simulink model "Motor_ctrl"  (R2025b)
settings: Solver=ode15s  StopTime=Tend_sim  FixedStep=Ts/10  MaxStep=Tstep  AbsTol=1e-3  EnableMultiTasking=on
InitFcn:
  | if ~exist('flagwp')
  |     tic
  |     init_sim
  | end
  | mex Motor_ctrl.c User_functions/Src/*.c
StopFcn:
  | % if ~exist('flagwp')
  |   elapsed_time=toc
  | % end
  | %plot_out_sim
values from neighbouring files (symbols this model uses):
  accel = 30000    [init_sim.m]
  Bm = 0.02    [init_sim.m]
  Clarke_inv = [1 0;-0.5 sqrt(3)/2;-0.5 -sqrt(3)/2]    [init_sim.m]
  Ctrl_strategy = 1    [init_sim.m]
  Ctrl_type = 3    [init_sim.m]
  dem = 1    [init_sim.m]
  dT = motorModel.SyreDrive.Converter.dT * 1e-6    [init_sim.m]
  EV_mode = 0    [init_sim.m]
  expC = motorModel.IronPMLossMap_dq.expC    [init_sim.m]
  expH = motorModel.IronPMLossMap_dq.expH    [init_sim.m]
  expPM = motorModel.IronPMLossMap_dq.expPM    [init_sim.m]
  Fd0 = interp2(motorModel.FluxMap_dq.Id,motorModel.FluxMap_dq.Iq,motorModel.FluxMap_dq.Fd,0,0)    [init_sim.m]
  fD_pu_norm = motorModel.FluxMapInv_dq.fD_pu_norm    [init_sim.m]
  fD_vct_max = motorModel.FluxMapInv_dq.fD_vct_max    [init_sim.m]
  fD_vct_ref = motorModel.FluxMapInv_dq.fD_vct_ref    [init_sim.m]
  Fm = interp2(Idd,Iqq,Fdd,0,0)    [init_sim.m]
  fQ_pu_norm = motorModel.FluxMapInv_dq.fQ_pu_norm    [init_sim.m]
  fQ_vct_max = motorModel.FluxMapInv_dq.fQ_vct_max    [init_sim.m]
  fQ_vct_ref = motorModel.FluxMapInv_dq.fQ_vct_ref    [init_sim.m]
  HS_ctrl = 1    [init_sim.m]
  Id_dqt = interpn(motorModel.FluxMapInv_dqt.dataF.Fd,motorModel.FluxMapInv_dqt.dataF.Fq,motorModel.FluxMapInv_dqt.dataF.th,motorModel.FluxMapInv_dqt.dataF.Id,Fd_dqt,Fq_dqt,th_dqt,'cubic')    [init_sim.m]
  Id_fe = motorModel.IronPMLossMap_dq.Id    [init_sim.m]
  iD_pu_norm = motorModel.FluxMapInv_dq.iD_pu_norm    [init_sim.m]
  idRef = interp1(abs(MTPA.id+1i*MTPA.iq),MTPA.id,i0)    [init_sim.m]
  InitIntg_d = Fm*cos(th0)    [init_sim.m]
  InitIntg_q = Fm*sin(th0)    [init_sim.m]
  inj_waveform = 1    [init_sim.m]
  Iq_dqt = interpn(motorModel.FluxMapInv_dqt.dataF.Fd,motorModel.FluxMapInv_dqt.dataF.Fq,motorModel.FluxMapInv_dqt.dataF.th,motorModel.FluxMapInv_dqt.dataF.Iq,Fd_dqt,Fq_dqt,th_dqt,'cubic')    [init_sim.m]
  Iq_fe = motorModel.IronPMLossMap_dq.Iq    [init_sim.m]
  iQ_pu_norm = motorModel.FluxMapInv_dq.iQ_pu_norm    [init_sim.m]
  iqRef = interp1(abs(MTPA.id+1i*MTPA.iq),MTPA.iq,i0)    [init_sim.m]
  IronLoss = 1    [init_sim.m]
  J = 2.7    [init_sim.m]
  motorModelType = motorModel.SyreDrive.modelSetup.motorModelType    [init_sim.m]
  n0 = motorModel.IronPMLossMap_dq.n0    [init_sim.m]
  nRef = 1000    [init_sim.m]
  p = motorModel.data.p    [init_sim.m]
  Pfe_c = motorModel.IronPMLossMap_dq.Pfes_c + motorModel.IronPMLossMap_dq.Pfer_c    [init_sim.m]
  Pfe_h = motorModel.IronPMLossMap_dq.Pfes_h + motorModel.IronPMLossMap_dq.Pfer_h    [init_sim.m]
  Ppm = motorModel.IronPMLossMap_dq.Ppm    [init_sim.m]
  Quad_Maps = 2    [init_sim.m]
  Rs = motorModel.data.Rs    [init_sim.m]
  SS_on = 1    [init_sim.m]
  T0 = interp2(motorModel.FluxMap_dq.Id,motorModel.FluxMap_dq.Iq,motorModel.FluxMap_dq.T,idRef,iqRef)    [init_sim.m]
  T_dqt = interpn(motorModel.FluxMapInv_dqt.dataF.Fd,motorModel.FluxMapInv_dqt.dataF.Fq,motorModel.FluxMapInv_dqt.dataF.th,motorModel.FluxMapInv_dqt.dataF.T,Fd_dqt,Fq_dqt,th_dqt,'cubic')    [init_sim.m]
  Tf = 6    [init_sim.m]
  th0 = 0    [init_sim.m]
  th_max = max(motorModel.FluxMapInv_dqt.dataF.th,[],'all')    [init_sim.m]
  th_min = min(motorModel.FluxMapInv_dqt.dataF.th,[],'all')    [init_sim.m]
  Ts = 1/motorModel.SyreDrive.Converter.fPWM    [init_sim.m]
  Tv = 7.1e-6    (= 7.1e-06)    [init_sim.m]
  VDC = motorModel.data.Vdc    [init_sim.m]
undefined symbols (not defined in the file or in its folder): ACloss, eMotor, interpn, J_rot, magnitude, n0_inv
libraries: nesl_utility x31, fl_lib x26, simulink x10, ee_lib x8, eeTransforms x1
(part 1 of 4)
settings Model: SimulationMode=accelerator  Creator=work  LastModifiedBy=Simone Ferrari
settings SolverCC: ZeroCrossAlgorithm=Adaptive  AlgebraicLoopSolver=TrustRegion
settings DataIOCC: FinalStateName=xFinalSim  InitialState=xFinalSim  SaveFormat=Array  SignalLoggingSaveFormat=ModelDataLogs  SaveOutput=off  SignalLogging=off  DSMLogging=off  TimeSaveName=time  SignalLoggingName=sigsOut
settings OptimizationCC: BlockReduction=off  BooleanDataType=off  ExpressionDepthLimit=2147483647.0  InitFltsAndDblsToZero=on  LifeSpan=inf
settings DebuggingCC: SaveWithParameterizedLinksMsg=none  SignalResolutionControl=TryResolveAllWithWarning  IgnoredZcDiagnostic=none  MultiTaskDSMMsg=warning  MultiTaskCondExecSysMsg=none  FcnCallInpInsideContextMsg=warning  UnconnectedInputMsg=warning  UnconnectedOutputMsg=warning  UnconnectedLineMsg=warning  StateNameClashWarn=warning  SFUnexpectedBacktrackingDiag=warning  SFNoUnconditionalDefaultTransitionDiag=warning  SFExecutionAtInitializationDiag=none  ArithmeticOperatorsInVariantConditions=warning
settings HardwareCC: ProdBitPerPointer=32.0  ProdBitPerSizeT=32.0  ProdBitPerPtrDiffT=32.0  ProdLargestAtomicFloat=None  ProdIntDivRoundTo=Undefined  ProdEndianess=Unspecified  ProdWordSize=32.0  ProdHWDeviceType=32-bit Generic  TargetBitPerPointer=64.0  TargetBitPerSizeT=64.0  TargetBitPerPtrDiffT=64.0  TargetLongLongMode=on  TargetIntDivRoundTo=Zero  TargetEndianess=LittleEndian  TargetWordSize=64.0  TargetHWDeviceType=MATLAB Host  ProdEqTarget=off
settings ModelReferenceCC: EnableRefExpFcnMdlSchedulingChecks=on
settings SFSimCC: SimUseLocalCustomCode=off  CustomCodeUndefinedFunction=UseInterfaceOnly
settings RTWCC: RTWUseLocalCustomCode=off  GPUComputeCapability=3.5  DLArmComputeVersion=19.05
settings CodeAppCC: StateflowObjectComments=on
settings GRTTargetCC: TargetFcnLib=ansi_tfl_tmw.mat  TargetLangStandard=C89/C90 (ANSI)  CombineOutputUpdateFcns=off  GRTInterface=on
settings ConfigComp: CovMetricSettings=dw  CovSaveCumulativeToWorkspaceVar=on  CovSaveSingleToWorkspaceVar=on  CovExternalEMLEnable=off  CovSFcnEnable=off

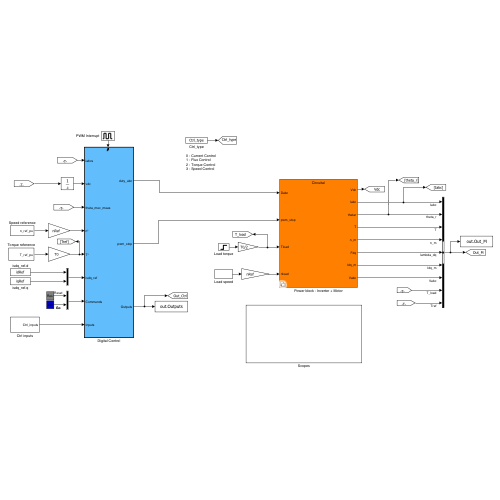
[thumbnail: Simulink's stored preview of the top-level diagram]
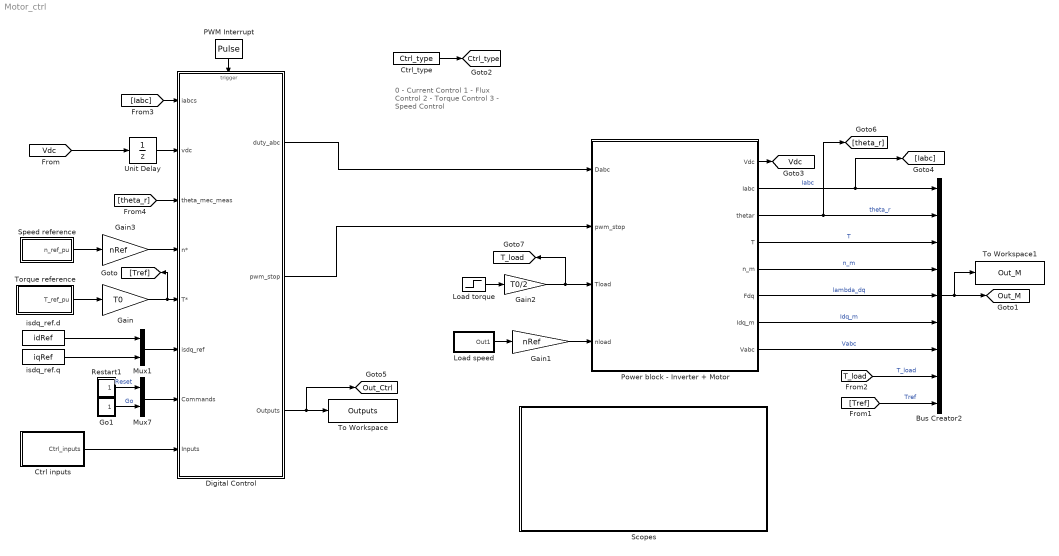
== system Motor_ctrl ==
  note: 0 - Current Control
      | 1 - Flux Control
      | 2 - Torque Control
      | 3 - Speed Control
  Bus Creator2 : BusCreator  Inputs=9
  Ctrl inputs : Subsystem
  Ctrl_type : Constant  Value=Ctrl_type
  Digital Control : Subsystem  TreatAsAtomicUnit=on
  Gain : Gain  Gain=T0
  Gain1 : Gain  Gain=nRef
  Gain2 : Gain  Gain=T0/2
  Gain3 : Gain  Gain=nRef
  Go1 : Subsystem
  Load speed : Subsystem
  Load torque : Step  Time=0.6  SampleTime=0
  Mux1 : Mux  Inputs=2
  Mux7 : Mux  Inputs=2
  PWM Interrupt : DiscretePulseGenerator  PulseType=Time based  Period=Ts  PulseWidth=50
  Power block - Inverter + Motor : Subsystem  Variant=on
  Restart1 : Subsystem
  Scopes : Subsystem
  Speed reference : Subsystem
  To Workspace : ToWorkspace  VariableName=Outputs  SaveFormat=Timeseries  SampleTime=-1
      settings: Decimation=n_dec
  To Workspace1 : ToWorkspace  VariableName=Out_M  SaveFormat=Timeseries  SampleTime=-1
      settings: Decimation=n_dec
  Torque reference : Subsystem
  Unit Delay : UnitDelay  SampleTime=-1
  isdq_ref.d : Constant  Value=idRef
  isdq_ref.q : Constant  Value=iqRef
  tag scope: Ctrl_type=global, Out_Ctrl=global, Out_M=global, T_load=global, Vdc=global
  wires:
  Gain/1 -> [Tref], Digital Control/5(T*)
  Digital Control/2(pwm_stop) -> Power block - Inverter + Motor/2(pwm_stop)
  Unit Delay/1 -> Digital Control/2(vdc)
  isdq_ref.d/1 -> Mux1/1
  Restart1/1(Res) -> Mux7/1  "Reset"
  isdq_ref.q/1 -> Mux1/2
  PWM Interrupt/1 -> Digital Control/Trigger
  Gain3/1 -> Digital Control/4(n*)
  Digital Control/3(Outputs) -> [Out_Ctrl], To Workspace/1
  Digital Control/1(duty_abc) -> Power block - Inverter + Motor/1(Dabc)
  Mux7/1 -> Digital Control/7(Commands)
  Ctrl_type/1 -> [Ctrl_type]
  Gain2/1 -> Power block - Inverter + Motor/3(Tload), [T_load]
  Load torque/1 -> Gain2/1
  Mux1/1 -> Digital Control/6(isdq_ref)
  Go1/1(Go) -> Mux7/2  "Go"
  Speed reference/1(n_ref_pu) -> Gain3/1
  [T_load] -> Bus Creator2/8  "T_load"
  Power block - Inverter + Motor/2(Iabc) -> Bus Creator2/1, [Iabc]  "Iabc"
  Power block - Inverter + Motor/7(Idq_m) -> Bus Creator2/6  "Idq_m"
  Power block - Inverter + Motor/5(n_m) -> Bus Creator2/4  "n_m"
  Power block - Inverter + Motor/3(thetar) -> Bus Creator2/2, [theta_r]  "theta_r"
  Power block - Inverter + Motor/4(T) -> Bus Creator2/3  "T"
  [Tref] -> Bus Creator2/9  "Tref"
  Bus Creator2/1 -> To Workspace1/1, [Out_M]
  Power block - Inverter + Motor/6(Fdq) -> Bus Creator2/5  "lambda_dq"
  Power block - Inverter + Motor/8(Vabc) -> Bus Creator2/7  "Vabc"
  Gain1/1 -> Power block - Inverter + Motor/4(nload)
  Torque reference/1(T_ref_pu) -> Gain/1
  Ctrl inputs/1(Ctrl_inputs) -> Digital Control/8(Inputs)
  Power block - Inverter + Motor/1(Vdc) -> [Vdc]
  [Vdc] -> Unit Delay/1
  [Iabc] -> Digital Control/1(iabcs)
  [theta_r] -> Digital Control/3(theta_mec_meas)
  Load speed/1(Out1) -> Gain1/1

== system Motor_ctrl/Ctrl inputs ==
  Constant1 : Constant  Value=Fm
  Constant10 : Constant  Value=Quad_Maps
  Constant2 : Constant  Value=th0
  Constant3 : Constant  Value=Ctrl_strategy
  Constant5 : Constant  Value=SS_on
  Constant6 : Constant  Value=inj_waveform
  Constant7 : Constant  Value=HS_ctrl
  Constant8 : Constant  Value=dem
  Constant9 : Constant  Value=accel
  Mux9 : Mux  Inputs=10
  Ctrl_inputs : Outport
  wires:
  Constant7/1 -> Mux9/5
  Constant10/1 -> Mux9/8
  Constant3/1 -> Mux9/2
  Constant6/1 -> Mux9/3
  Constant1/1 -> Mux9/9
  Constant8/1 -> Mux9/4
  Constant9/1 -> Mux9/7
  Constant2/1 -> Mux9/10
  Constant5/1 -> Mux9/6
  [Ctrl_type] -> Mux9/1
  Mux9/1 -> Ctrl_inputs/1

== system Motor_ctrl/Digital Control ==
  iabcs : Inport
  vdc : Inport  Port=2
  theta_mec_meas : Inport  Port=3
  n* : Inport  Port=4
  T* : Inport  Port=5
  isdq_ref : Inport  Port=6
  Commands : Inport  Port=7
  Inputs : Inport  Port=8
  Trigger : TriggerPort  VariantControl=(inherit)
  Bus Creator : BusCreator  Inputs=42
  Control S-Function : S-Function  FunctionName=Motor_ctrl  SFunctionDeploymentMode=off  EnableBusSupport=off
  Demux1 : Demux  Outputs=2
  Demux2 : Demux  Outputs=45
  Mux : Mux  Inputs=9
  Mux1 : Mux  Inputs=3
  Unit Delay : UnitDelay  SampleTime=-1
  duty_abc : Outport
  pwm_stop : Outport  Port=2
  Outputs : Outport  Port=3
  wires:
  Mux/1 -> Control S-Function/1
  vdc/1 -> Mux/2
  theta_mec_meas/1 -> Mux/3
  Control S-Function/1 -> Unit Delay/1
  n*/1 -> Mux/4
  Mux1/1 -> Bus Creator/1, duty_abc/1  "duty_abc"
  Demux1/1 -> Mux/7  "Reset"
  Demux1/2 -> Mux/8  "Go"
  Commands/1 -> Demux1/1
  isdq_ref/1 -> Mux/6
  Unit Delay/1 -> Demux2/1
  Demux2/1 -> Mux1/1  "duty_a"
  Demux2/2 -> Mux1/2  "duty_b"
  Demux2/3 -> Mux1/3  "duty_c"
  Demux2/4 -> pwm_stop/1
  T*/1 -> Mux/5
  Inputs/1 -> Mux/9
  Bus Creator/1 -> Outputs/1
  Demux2/34 -> Bus Creator/31  "pos_err_HS"
  Demux2/33 -> Bus Creator/30  "pos_err_LS"
  Demux2/32 -> Bus Creator/29  "pos_err_real"
  Demux2/31 -> Bus Creator/28  "pos_err"
  Demux2/30 -> Bus Creator/27  "theta_elt_meas"
  Demux2/29 -> Bus Creator/26  "iC"
  Demux2/28 -> Bus Creator/25  "iB"
  Demux2/27 -> Bus Creator/24  "iA"
  Demux2/26 -> Bus Creator/23  "ldq"
  Demux2/25 -> Bus Creator/22  "lq"
  Demux2/24 -> Bus Creator/21  "ld"
  Demux2/23 -> Bus Creator/20  "n_ctrl"
  Demux2/22 -> Bus Creator/19  "theta_elt"
  Demux2/21 -> Bus Creator/18  "T_ext"
  Demux2/20 -> Bus Creator/17  "lambdaQ_CM"
  Demux2/18 -> Bus Creator/15  "lambdaQ"
  Demux2/19 -> Bus Creator/16  "lambdaD_CM"
  Demux2/17 -> Bus Creator/14  "lambdaD"
  Demux2/16 -> Bus Creator/13  "T_elt"
  Demux2/15 -> Bus Creator/12  "f_w"
  Demux2/14 -> Bus Creator/11  "iq"
  Demux2/13 -> Bus Creator/10  "iq_ref"
  Demux2/12 -> Bus Creator/9  "id"
  Demux2/11 -> Bus Creator/8  "id_ref"
  Demux2/10 -> Bus Creator/7  "isbeta"
  Demux2/9 -> Bus Creator/6  "isalpha"
  Demux2/8 -> Bus Creator/5  "vq_ref"
  Demux2/7 -> Bus Creator/4  "vd_ref"
  Demux2/6 -> Bus Creator/3  "wr"
  Demux2/5 -> Bus Creator/2  "wr_ref"
  iabcs/1 -> Mux/1
  Demux2/35 -> Bus Creator/32  "lambda_ref"
  Demux2/36 -> Bus Creator/33  "lambda_fbk"
  Demux2/37 -> Bus Creator/34  "iqs_ref"
  Demux2/38 -> Bus Creator/35  "iqs_fbk"
  Demux2/39 -> Bus Creator/36  "delta_max"
  Demux2/40 -> Bus Creator/37  "delta_fbk"
  Demux2/41 -> Bus Creator/38  "i_MTPV"
  Demux2/42 -> Bus Creator/39  "iqs_Lim"
  Demux2/43 -> Bus Creator/40  "vds_ref"
  Demux2/44 -> Bus Creator/41  "vqs_ref"
  Demux2/45 -> Bus Creator/42  "State"

== system Motor_ctrl/Go1 ==
  GO_Down : Step  Time=0.01+4*Ts  SampleTime=0
  GO_Up : Step  Time=0.01  SampleTime=0
  Subtract : Sum  Inputs=+-
  Go : Outport
  wires:
  Subtract/1 -> Go/1
  GO_Up/1 -> Subtract/1
  GO_Down/1 -> Subtract/2

== system Motor_ctrl/Load speed ==
  LoadSpeedRamp : simulink/Sources/Ramp  slope=20  start=0.2  InitialOutput=0
  LoadSpeedSat : Saturate  UpperLimit=1  LowerLimit=-1
  Out1 : Outport
  wires:
  LoadSpeedRamp/1 -> LoadSpeedSat/1
  LoadSpeedSat/1 -> Out1/1

== system Motor_ctrl/Power block - Inverter + Motor ==
  note: 1) Add Subsystem or Model blocks as valid variant choices.
      | 2) You cannot connect blocks at this level. At simulation, connectivity is automatically
      | determined, based on the active variant and port name matching.
  Dabc : Inport
  pwm_stop : Inport  Port=2
  Tload : Inport  Port=3
  nload : Inport  Port=4
  Circuital : Subsystem  VariantControl=strcmp(motorModelType,'Controlled Current Generators (CCG)') || strcmp(motorModelType,'SimScape FEM-based PMSM')
  Noncircuital : Subsystem  VariantControl=strcmp(motorModelType,'Non-Circuital Model (FM)')
  Vdc : Outport
  Iabc : Outport  Port=2
  thetar : Outport  Port=3
  T : Outport  Port=4
  n_m : Outport  Port=5
  Fdq : Outport  Port=6
  Idq_m : Outport  Port=7
  Vabc : Outport  Port=8

== system Motor_ctrl/Restart1 ==
  "DOWN " : Step  Time=10e-3+4*Ts  SampleTime=0
  Subtract : Sum  Inputs=+-
  "UP " : Step  Time=10e-3  SampleTime=0
  Res : Outport
  wires:
  "UP "/1 -> Subtract/1
  "DOWN "/1 -> Subtract/2
  Subtract/1 -> Res/1

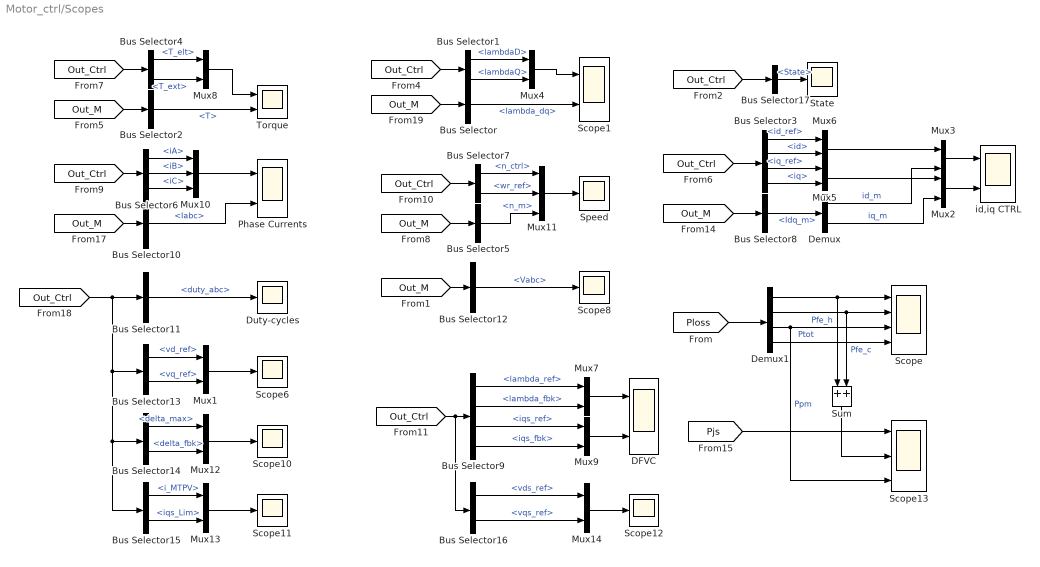
== system Motor_ctrl/Scopes ==
  Bus Selector : BusSelector  OutputSignals=lambda_dq
  Bus Selector1 : BusSelector  OutputSignals=lambdaD,lambdaQ
  Bus Selector10 : BusSelector  OutputSignals=Iabc
  Bus Selector11 : BusSelector  OutputSignals=duty_abc
  Bus Selector12 : BusSelector  OutputSignals=Vabc
  Bus Selector13 : BusSelector  OutputSignals=vd_ref,vq_ref
  Bus Selector14 : BusSelector  OutputSignals=delta_max,delta_fbk
  Bus Selector15 : BusSelector  OutputSignals=i_MTPV,iqs_Lim
  Bus Selector16 : BusSelector  OutputSignals=vds_ref,vqs_ref
  Bus Selector17 : BusSelector  OutputSignals=State
  Bus Selector2 : BusSelector  OutputSignals=T
  Bus Selector3 : BusSelector  OutputSignals=id_ref,id,iq_ref,iq
  Bus Selector4 : BusSelector  OutputSignals=T_elt,T_ext
  Bus Selector5 : BusSelector  OutputSignals=n_m
  Bus Selector6 : BusSelector  OutputSignals=iA,iB,iC
  Bus Selector7 : BusSelector  OutputSignals=n_ctrl,wr_ref
  Bus Selector8 : BusSelector  OutputSignals=Idq_m
  Bus Selector9 : BusSelector  OutputSignals=lambda_ref,lambda_fbk,iqs_ref,iqs_fbk
  DFVC : Scope  NumInputPorts=2
      settings: ActiveDisplayYMinimum=-0.016936566680669781  ActiveDisplayYMaximum=0.15242910012602806
  Demux : Demux  Outputs=2
  Demux1 : Demux
  Duty-cycles : Scope
      settings: ActiveDisplayYMinimum=-0.14215802685897236  ActiveDisplayYMaximum=1.1077597187312376
  Mux{1..9,12..14} (12 alike) : Mux  Inputs=2
  Mux10 : Mux  Inputs=3
  Mux11 : Mux  Inputs=3
  Phase Currents : Scope  NumInputPorts=2
      settings: ActiveDisplayYMinimum=-1311.5522096192847  ActiveDisplayYMaximum=1325.5199197219822
  Scope : Scope  NumInputPorts=4
      settings: ActiveDisplayYMinimum=-1  ActiveDisplayYMaximum=1
  Scope1 : Scope  NumInputPorts=2
      settings: ActiveDisplayYMinimum=-1  ActiveDisplayYMaximum=1
  Scope{6,8,10..12} (5 alike) : Scope
      Scope10 settings: ActiveDisplayYMinimum=-1  ActiveDisplayYMaximum=1
      Scope11 settings: ActiveDisplayYMinimum=-125.78182983398435  ActiveDisplayYMaximum=1132.0364685058594
      Scope12 settings: ActiveDisplayYMinimum=-230.93904685974121  ActiveDisplayYMaximum=230.93997764587402
      Scope6 settings: ActiveDisplayYMinimum=-287.14855575561523  ActiveDisplayYMaximum=243.69842147827148
  Scope13 : Scope  NumInputPorts=3
      settings: ActiveDisplayYMinimum=-1  ActiveDisplayYMaximum=1
  Speed : Scope
      settings: ActiveDisplayYMinimum=-450.47500610351551  ActiveDisplayYMaximum=4054.2750549316406  DataLoggingVariableName=ScopeData2
  State : Scope
      settings: ActiveDisplayYMinimum=-0.37499999999999989  ActiveDisplayYMaximum=3.375  DataLoggingVariableName=ScopeData5
  Sum : Sum
  Torque : Scope  NumInputPorts=2
      settings: ActiveDisplayYMinimum=-62.272152420628927  ActiveDisplayYMaximum=554.91717274463247
  id,iq CTRL : Scope  NumInputPorts=2
      settings: ActiveDisplayYMinimum=-1103.0936021552059  ActiveDisplayYMaximum=934.58880271777161
  wires:
  Bus Selector3/2 -> Mux6/2  "<id>"
  [Out_M] -> Bus Selector2/1
  Mux4/1 -> Scope1/1
  [Out_M] -> Bus Selector12/1
  Bus Selector/1 -> Scope1/2  "<lambda_dq>"
  Bus Selector10/1 -> Phase Currents/2  "<Iabc>"
  Bus Selector1/2 -> Mux4/2  "<lambdaQ>"
  Bus Selector3/3 -> Mux5/1  "<iq_ref>"
  Bus Selector3/4 -> Mux5/2  "<iq>"
  Bus Selector4/1 -> Mux8/1  "<T_elt>"
  Mux6/1 -> Mux3/1
  Demux/1 -> Mux3/2  "id_m"
  [Out_M] -> Bus Selector5/1
  Bus Selector1/1 -> Mux4/1  "<lambdaD>"
  Bus Selector6/3 -> Mux10/3  "<iC>"
  Bus Selector6/2 -> Mux10/2  "<iB>"
  [Out_Ctrl] -> Bus Selector6/1
  [Out_Ctrl] -> Bus Selector1/1
  [Out_Ctrl] -> Bus Selector4/1
  Mux5/1 -> Mux2/1
  Bus Selector6/1 -> Mux10/1  "<iA>"
  [Out_Ctrl] -> Bus Selector7/1
  Mux10/1 -> Phase Currents/1
  [Out_M] -> Bus Selector8/1
  Bus Selector3/1 -> Mux6/1  "<id_ref>"
  [Out_Ctrl] -> Bus Selector3/1
  [Out_M] -> Bus Selector10/1
  Bus Selector12/1 -> Scope8/1  "<Vabc>"
  Mux8/1 -> Torque/1
  Bus Selector8/1 -> Demux/1  "<Idq_m>"
  Demux/2 -> Mux2/2  "iq_m"
  Bus Selector11/1 -> Duty-cycles/1  "<duty_abc>"
  Mux3/1 -> id,iq CTRL/1
  Mux2/1 -> id,iq CTRL/2
  [Out_M] -> Bus Selector/1
  Mux11/1 -> Speed/1
  Demux1/1 -> Sum/1, Scope/1  "Pfe_h"
  Demux1/2 -> Sum/2, Scope/2  "Pfe_c"
  Demux1/4 -> Scope/4  "Ptot"
  Demux1/3 -> Scope13/3, Scope/3  "Ppm"
  Bus Selector2/1 -> Torque/2  "<T>"
  Bus Selector4/2 -> Mux8/2  "<T_ext>"
  Mux1/1 -> Scope6/1
  Bus Selector13/1 -> Mux1/1  "<vd_ref>"
  Bus Selector13/2 -> Mux1/2  "<vq_ref>"
  [Ploss] -> Demux1/1
  [Out_Ctrl] -> Bus Selector16/1, Bus Selector9/1
  Mux7/1 -> DFVC/1
  Bus Selector9/1 -> Mux7/1  "<lambda_ref>"
  Bus Selector9/2 -> Mux7/2  "<lambda_fbk>"
  Bus Selector9/3 -> Mux9/1  "<iqs_ref>"
  Bus Selector9/4 -> Mux9/2  "<iqs_fbk>"
  Mux9/1 -> DFVC/2
  Bus Selector14/2 -> Mux12/2  "<delta_fbk>"
  Mux12/1 -> Scope10/1
  Bus Selector14/1 -> Mux12/1  "<delta_max>"
  Mux13/1 -> Scope11/1
  Bus Selector15/2 -> Mux13/2  "<iqs_Lim>"
  Bus Selector15/1 -> Mux13/1  "<i_MTPV>"
  Bus Selector7/1 -> Mux11/1  "<n_ctrl>"
  Bus Selector7/2 -> Mux11/2  "<wr_ref>"
  Bus Selector5/1 -> Mux11/3  "<n_m>"
  Bus Selector16/2 -> Mux14/2  "<vqs_ref>"
  Mux14/1 -> Scope12/1
  Bus Selector16/1 -> Mux14/1  "<vds_ref>"
  [Out_Ctrl] -> Bus Selector15/1, Bus Selector14/1, Bus Selector13/1, Bus Selector11/1
  [Pjs] -> Scope13/1
  Sum/1 -> Scope13/2
  [Out_Ctrl] -> Bus Selector17/1
  Bus Selector17/1 -> State/1  "<State>"

== system Motor_ctrl/Speed reference ==
  RefSpeedRamp : simulink/Sources/Ramp  slope=20  start=0.2  InitialOutput=0
  RefSpeedRampSat : Saturate  UpperLimit=1  LowerLimit=-1
  n_ref_pu : Outport
  wires:
  RefSpeedRampSat/1 -> n_ref_pu/1
  RefSpeedRamp/1 -> RefSpeedRampSat/1

== system Motor_ctrl/Torque reference ==
  Constant4 : Constant  Value=EV_mode
  EV mode Vs test bench : Switch  Criteria=u2 > Threshold  Threshold=0.5  SaturateOnIntegerOverflow=off  InputSameDT=off
  Step : Step  Time=0.05  SampleTime=0
  Step1 : Step  Time=0.15  SampleTime=0
  Step2 : Step  Time=0.8  After=-2  SampleTime=0
  Sum : Sum
  T_ref_pu : Outport
  wires:
  Constant4/1 -> EV mode Vs test bench/2
  Step/1 -> EV mode Vs test bench/1
  EV mode Vs test bench/1 -> T_ref_pu/1
  Sum/1 -> EV mode Vs test bench/3
  Step2/1 -> Sum/2
  Step1/1 -> Sum/1

== system Motor_ctrl/Power block - Inverter + Motor/Circuital ==
  Dabc : Inport
  pwm_stop : Inport  Port=2
  Tload : Inport  Port=3
  nload : Inport  Port=4
  Inverter Model : Subsystem
  Motor model : Subsystem  Variant=on
  Vdc : Outport
  Iabc : Outport  Port=2
  thetar : Outport  Port=3
  T : Outport  Port=4
  n_m : Outport  Port=5
  Fdq : Outport  Port=6
  Idq_m : Outport  Port=7
  Vabc : Outport  Port=8
  wires:
  Inverter Model/1(Vdc) -> Vdc/1
  Tload/1 -> Motor model/1(Tload)
  nload/1 -> Motor model/2(nload)
  Dabc/1 -> Inverter Model/1(Dabc)
  pwm_stop/1 -> Inverter Model/2(pwm_stop)
  Motor model/1(Iabc) -> Inverter Model/3(Iabc), Iabc/1  "Iabc"
  Motor model/2(thetar) -> thetar/1  "theta_r"
  Motor model/3(T) -> T/1  "T"
  Motor model/4(n_m) -> n_m/1  "n_m"
  Motor model/5(Fdq) -> Fdq/1  "lambda_dq"
  Motor model/6(Idq_m) -> Idq_m/1  "Idq_m"
  Motor model/7(Vabc) -> Vabc/1  "Vabc"
  connections:
  Inverter Model/RConn1 -- Motor model/LConn1
  Inverter Model/RConn2 -- Motor model/LConn2
  Inverter Model/RConn3 -- Motor model/LConn3

== system Motor_ctrl/Power block - Inverter + Motor/Noncircuital ==
  Dabc : Inport
  pwm_stop : Inport  Port=2
  Tload : Inport  Port=3
  nload : Inport  Port=4
  FM : Subsystem
  Inverter Model : Subsystem  VariantControl=Choice
  Vdc : Outport
  Iabc : Outport  Port=2
  thetar : Outport  Port=3
  T : Outport  Port=4
  n_m : Outport  Port=5
  Fdq : Outport  Port=6
  Idq_m : Outport  Port=7
  Vabc : Outport  Port=8
  wires:
  FM/4(n_m) -> n_m/1  "n_m"
  FM/1(Iabc) -> Iabc/1, Inverter Model/3(Iabc)  "Iabc"
  FM/3(Tm) -> T/1  "T_m"
  FM/5(Fdq) -> Fdq/1  "lambda_dq"
  FM/2(thetar) -> thetar/1  "theta_r"
  FM/6(Idq_m) -> Idq_m/1  "Idq_m"
  pwm_stop/1 -> Inverter Model/2(pwm_stop)
  Tload/1 -> FM/1(Tload)
  Dabc/1 -> Inverter Model/1(Dabc)
  FM/7(Vabc) -> Vabc/1  "Vabc"
  nload/1 -> FM/2(nload)
  Inverter Model/1(Vdc) -> Vdc/1
  Inverter Model/2(Va) -> FM/3(A)
  Inverter Model/3(Vb) -> FM/4(B)
  Inverter Model/4(Vc) -> FM/5(C)

== system Motor_ctrl/Power block - Inverter + Motor/Circuital/Inverter Model ==
  Dabc : Inport
  pwm_stop : Inport  Port=2
  Iabc : Inport  Port=3
  " " : Fcn  Expr=1-u(1)
  Converter (Three-Phase) : ee_lib/Semiconductors & Converters/Converters/Converter (Three-Phase)  port_option=ee.enum.threePhasePort.expanded  fidelity_option=ee.enum.converters.fidelity.detailed  device_type=ee.enum.converters.switchingdevice.ideal  showThermalPort=false  K=0  Vth=0.001 V  Vgt=1 V  Vgt_off=-1 V  Ih=1 A  Vf=0.001 V  Ron=Rd Ohm  Rds=0.001 Ohm  Goff=1e-4 1/Ohm  Eon_scalar=22.86e-3 J  Eoff_scalar=17.14e-3 J  Eoff_natural_commutation=10e-3 J  Voff=300 V  Iout_scalar=600 A  onCurrentMeasDelay=0 s  useCurrentFromPreviousCycle=false  useVoltageFromPreviousCycle=false  diode_param=ee.enum.converters.protectiondiode.nodynamics  diode_Vf=0.8 V  diode_Ron=1e-4 Ohm  diode_Goff=1e-5 1/Ohm  diode_C=50 nF  diode_iRM=-235 A  diode_iF=300 A  diode_idot=-50 A/us  diode_trr_param=ee.enum.converters.diodetrr.trr_factor  diode_trr_factor=3  diode_trr=15 us  diode_Qrr=1500 s*uA  diode_rec_loss_model=ee.enum.diode.reverseRecoveryModel.fixed  diode_ErecVal=0 J  diode_scaleWithIandV=false  diode_ErecMat=zeros(2, 3) J  diode_TjrecVec=[298.15, 398.15] K  diode_IfrecVec=[.1, 1, 10] A  diode_IrecVal=10 A  diode_VrecVal=10 V  diode_tFilter=1 / 1000 / 100 s  thermal_network_parameterization=ee.enum.thermalNetworkTopology.external  Rth=[.08, .5] K/W  Rth_Cauer=[.08, .1, .5] K/W  Rth_Foster=[.08, .14, .22, .16] K/W  thermal_mass_parameterization=ee.enum.thermalNetwork.timeconstant  thermal_mass=[.01, .5] J/K  thermal_mass_Cauer=[.01, .1, .5] J/K  thermal_mass_Foster=[.001, .005, .05, .5] J/K  thermal_time_constant=[.001, .2] s  thermal_time_constant_Cauer=[.001, .1, .2] s  thermal_time_constant_Foster=[7e-05, .0007, .01, .08] s  thermal_mass_initial_temperatures=[25, 25] degC  thermal_mass_initial_temperatures_Cauer=[25, 25, 25] degC  junction_thermal_mass=0.01 J/K  Tvec_initial_Foster=[25, 25, 25, 25] degC  snubber_type=ee.enum.converters.snubber.exclude  Cs=1e-7 F  Rs=0.1 Ohm  Vce_loss=[0, 150, 300] V
  Demux : Demux  Outputs=6
  Electrical Reference : fl_lib/Electrical/Electrical Elements/Electrical Reference
  Inverter Commands : Subsystem  Variant=on
  PS-Simulink Converter : nesl_utility/PS-Simulink Converter  PhysicalDomain=network_engine_domain  SubClassName=ps_output  LeftPortType=input  RightPortType=output  PseudoPeriodic=off  Frequencies=[]  VectorFormat=1-D array  Unit=inherit  AffineConversion=off
  Simulink-PS Converter{,1..5} (6 alike) : nesl_utility/Simulink-PS Converter  PhysicalDomain=network_engine_domain  SubClassName=ps_input  LeftPortType=input  RightPortType=output  PseudoPeriodic=off  Frequencies=[]  NoiseDistribution=none  NoiseParameters=[]  Unit=1  AffineConversion=off  FilteringAndDerivatives=provide  SimscapeFilterOrder=1  InputFilterTimeConstant=0.001  UdotUserProvided=0
  Six-Pulse Gate Multiplexer : ee_lib/Semiconductors & Converters/Converters/Six-Pulse Gate Multiplexer  port_option=ee.enum.controlport.ps
  Solver Configuration : nesl_utility/Solver Configuration  PhysicalDomain=network_engine_domain  SubClassName=solver  LeftPortType=input  RightPortType=generic  Tones=[]  Harmonics=[]  SimulateNoise=off  Profile=off  UseLocalSampling=off  EnableSwitchedLinearOptims=on  FrequencyDomain=off  UseCCode=off  RelTol=0.001  AbsTol=1e-06  MinStep=1e-09  ToWorkspace=off  RevertToSquareIcSolve=off  NumHomotopyIterations=100  PhasorMode=off  PhasorModeNumHarmonics=1  ConsistencySolver=NEWTON_FTOL  CanonicalOrdering=UNORDERED  OptimizeIntermediates=UNOPTIMIZED  IndexReductionMethod=DerivativeReplacement  DoDC=off  ResidualTolerance=1e-09  ConsistencyTolSource=GLOBAL  ConsistencyAbsTol=0.001  ConsistencyRelTol=0.001  ConsistencyTolFactor=0.001  UseLocalSolver=off  LocalSolverChoice=NE_BACKWARD_EULER_ADVANCER  ResolveIndetEquations=on  FunctionEvalNumThread=1  LocalSolverSampleTime=Ts/10  DoFixedCost=off  MaxNonlinIter=3  MaxModeIter=2  ComputeImpulses=off  ImpulseIterations=2  LinearAlgebra=auto  LinearAlgebraNumThread=0  EquationFormulation=NE_TIME_EF  DelaysMemoryBudget=1024  AutomaticFiltering=on  FilteringTimeConstant=0.001  PartitionStorageMethod=AS_NEEDED  PartitionMemoryBudget=1024  PartitionMethod=ROBUST  MultibodyUseLocalSolver=off  MultibodyLocalSolverChoice=ODE1  MultibodyLocalSolverSampleTime=0.001
  Voltage Sensor : fl_lib/Electrical/Electrical Sensors/Voltage Sensor
  Voltage Source : ee_lib/Sources/Voltage Source  dc_voltage=0.5*VDC V  ac_voltage=0 V  ac_shift=0 rad  ac_frequency=60 Hz  noise_mode=0  PSD=0 V^2/Hz  sample_time=1e-3 s  repeatability=1  user_seed=0  auto_seed=676943032  i_specify=off  i_priority=None  i=0 A  i_nominal_specify=off  i_nominal_value=1  i_nominal_unit=A  v_specify=off  v_priority=None  v=0 V  v_nominal_specify=off  v_nominal_value=1  v_nominal_unit=V
  Voltage Source1 : ee_lib/Sources/Voltage Source  dc_voltage=0.5*VDC V  ac_voltage=0 V  ac_shift=0 rad  ac_frequency=60 Hz  noise_mode=0  PSD=0 V^2/Hz  sample_time=1e-3 s  repeatability=1  user_seed=0  auto_seed=4168664255  i_specify=off  i_priority=None  i=0 A  i_nominal_specify=off  i_nominal_value=1  i_nominal_unit=A  v_specify=off  v_priority=None  v=0 V  v_nominal_specify=off  v_nominal_value=1  v_nominal_unit=V
  A : PMIOPort  Side=Right
  B : PMIOPort  Port=2  Side=Right
  C : PMIOPort  Port=3  Side=Right
  Vdc : Outport
  wires:
  Iabc/1 -> Inverter Commands/3(iABC)
  Demux/3 -> Simulink-PS Converter2/1
  Demux/4 -> Simulink-PS Converter3/1
  Demux/5 -> Simulink-PS Converter4/1
  Demux/6 -> Simulink-PS Converter5/1
  Demux/1 -> Simulink-PS Converter/1
  Demux/2 -> Simulink-PS Converter1/1
  " "/1 -> Inverter Commands/2(Enable)
  PS-Simulink Converter/1 -> Vdc/1
  Dabc/1 -> Inverter Commands/1(Dabc)
  Inverter Commands/1(G) -> Demux/1
  pwm_stop/1 -> " "/1
  connections:
  Simulink-PS Converter/RConn1 -- Six-Pulse Gate Multiplexer/LConn1
  Simulink-PS Converter3/RConn1 -- Six-Pulse Gate Multiplexer/LConn4
  Solver Configuration/RConn1 -- Converter (Three-Phase)/RConn1 -- Voltage Sensor/LConn1 -- Voltage Source/LConn1
  Simulink-PS Converter4/RConn1 -- Six-Pulse Gate Multiplexer/LConn5
  Simulink-PS Converter2/RConn1 -- Six-Pulse Gate Multiplexer/LConn3
  Simulink-PS Converter1/RConn1 -- Six-Pulse Gate Multiplexer/LConn2
  Simulink-PS Converter5/RConn1 -- Six-Pulse Gate Multiplexer/LConn6
  Voltage Source1/RConn1 -- Converter (Three-Phase)/RConn2 -- Voltage Sensor/RConn2
  Voltage Source/RConn1 -- Voltage Source1/LConn1 -- Electrical Reference/LConn1
  Six-Pulse Gate Multiplexer/RConn1 -- Converter (Three-Phase)/LConn1
  A/RConn1 -- Converter (Three-Phase)/LConn2
  Converter (Three-Phase)/LConn3 -- B/RConn1
  Converter (Three-Phase)/LConn4 -- C/RConn1
  PS-Simulink Converter/LConn1 -- Voltage Sensor/RConn1

== system Motor_ctrl/Power block - Inverter + Motor/Circuital/Motor model ==
  note: 1) Add Subsystem or Model blocks as valid variant choices.
      | 2) You cannot connect blocks at this level. At simulation, connectivity is automatically
      | determined, based on the active variant and port name matching.
  Tload : Inport
  nload : Inport  Port=2
  CCG model : Subsystem  VariantControl=strcmp(motorModelType,'Controlled Current Generators (CCG)')
  SimScape FEM-based PMSM : Subsystem  VariantControl=strcmp(motorModelType,'SimScape FEM-based PMSM')
  A : PMIOPort  Side=Left
  B : PMIOPort  Port=2  Side=Left
  C : PMIOPort  Port=3  Side=Left
  Iabc : Outport
  thetar : Outport  Port=2
  T : Outport  Port=3
  n_m : Outport  Port=4
  Fdq : Outport  Port=5
  Idq_m : Outport  Port=6
  Vabc : Outport  Port=7

== system Motor_ctrl/Power block - Inverter + Motor/Noncircuital/FM ==
  Tload : Inport
  nload : Inport  Port=2
  A : Inport  Port=3
  B : Inport  Port=4
  C : Inport  Port=5
  Mechanical equations : Subsystem
  Motor Model : Subsystem
  Terminator1 : Terminator
  Unit Delay : UnitDelay  SampleTime=-1
  Iabc : Outport
  thetar : Outport  Port=2
  Tm : Outport  Port=3
  n_m : Outport  Port=4
  Fdq : Outport  Port=5
  Idq_m : Outport  Port=6
  Vabc : Outport  Port=7
  wires:
  Mechanical equations/3(thetar) -> Motor Model/2(theta_r), Unit Delay/1
  Motor Model/3(Fdq) -> Fdq/1
  B/1 -> Motor Model/4(B)
  Motor Model/1(Tm) -> Mechanical equations/2(Tm), Tm/1
  Mechanical equations/2(Pmec_out) -> Terminator1/1
  Unit Delay/1 -> thetar/1
  nload/1 -> Mechanical equations/3(RPM)
  Tload/1 -> Mechanical equations/1(Tload)
  Motor Model/5(Vabc) -> Vabc/1
  Mechanical equations/1(n_m) -> Motor Model/1(n_m), n_m/1
  Motor Model/2(Iabc) -> Iabc/1
  Motor Model/4(Idq_m) -> Idq_m/1
  C/1 -> Motor Model/5(C)
  A/1 -> Motor Model/3(A)

== system Motor_ctrl/Power block - Inverter + Motor/Noncircuital/Inverter Model ==
  Dabc : Inport
  pwm_stop : Inport  Port=2
  Iabc : Inport  Port=3
  " " : Fcn  Expr=1-u(1)
  Constant : Constant  Value=VDC
  Demux : Demux  Outputs=3
  Inverter Commands : Subsystem  Variant=on
  Vdc : Outport
  Va : Outport  Port=2
  Vb : Outport  Port=3
  Vc : Outport  Port=4
  wires:
  Iabc/1 -> Inverter Commands/3(iABC)
  pwm_stop/1 -> " "/1
  " "/1 -> Inverter Commands/2(Enable)
  Dabc/1 -> Inverter Commands/1(Dabc)
  Demux/3 -> Vc/1
  Demux/2 -> Vb/1
  Demux/1 -> Va/1
  Inverter Commands/1(Vabc) -> Demux/1
  Constant/1 -> Vdc/1

== system Motor_ctrl/Power block - Inverter + Motor/Circuital/Inverter Model/Inverter Commands ==
  note: 1) Add Subsystem or Model blocks as valid variant choices.
      | 2) You cannot connect blocks at this level. At simulation, connectivity is automatically
      | determined, based on the active variant and port name matching.
  Dabc : Inport
  Enable : Inport  Port=2
  iABC : Inport  Port=3
  Duty : Subsystem  VariantControl=InvModel==0
  PWM : Subsystem  VariantControl=InvModel==1
  G : Outport

== system Motor_ctrl/Power block - Inverter + Motor/Circuital/Motor model/CCG model ==
  Tload : Inport
  nload : Inport  Port=2
  Mechanical equations : Subsystem
  Motor Model : Subsystem
  A : PMIOPort  Side=Left
  B : PMIOPort  Port=2  Side=Left
  C : PMIOPort  Port=3  Side=Left
  Iabc : Outport
  thetar : Outport  Port=2
  T : Outport  Port=3
  n_m : Outport  Port=4
  Fdq : Outport  Port=5
  Idq_m : Outport  Port=6
  Vabc : Outport  Port=7
  wires:
  Mechanical equations/1(n_m) -> Motor Model/1(n_m), n_m/1
  Motor Model/3(Fdq) -> Fdq/1
  Motor Model/5(Vabc) -> Vabc/1
  Motor Model/4(Idq_m) -> Idq_m/1
  Motor Model/1(Te) -> Mechanical equations/2(Te)
  Motor Model/2(Iabc) -> Iabc/1
  Mechanical equations/2(thetar) -> thetar/1, Motor Model/2(theta_r)
  nload/1 -> Mechanical equations/3(RPM)
  Tload/1 -> Mechanical equations/1(Tload)
  Mechanical equations/3(T) -> T/1
  connections:
  B/RConn1 -- Motor Model/LConn2
  C/RConn1 -- Motor Model/LConn3
  A/RConn1 -- Motor Model/LConn1

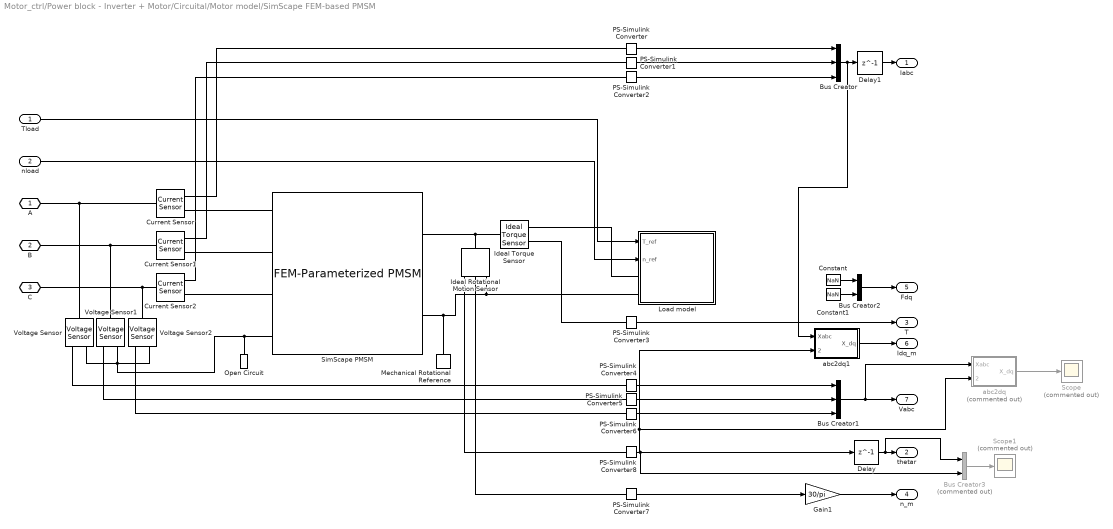
== system Motor_ctrl/Power block - Inverter + Motor/Circuital/Motor model/SimScape FEM-based PMSM ==
  Tload : Inport
  nload : Inport  Port=2
  Bus Creator : BusCreator  Inputs=3
  Bus Creator1 : BusCreator  Inputs=3
  Bus Creator2 : BusCreator  Inputs=2
  Bus Creator3 : BusCreator  Commented=on  Inputs=2
  Constant : Constant  Value=NaN
  Constant1 : Constant  Value=NaN
  Current Sensor : fl_lib/Electrical/Electrical Sensors/Current Sensor
  Current Sensor1 : fl_lib/Electrical/Electrical Sensors/Current Sensor
  Current Sensor2 : fl_lib/Electrical/Electrical Sensors/Current Sensor
  Delay : Delay  DelayLength=1  InitialCondition=0
  Delay1 : Delay  DelayLength=1  InitialCondition=0
  Gain1 : Gain  Gain=30/pi
  Ideal Rotational Motion Sensor : fl_lib/Mechanical/Mechanical Sensors/Ideal Rotational Motion Sensor  reference=foundation.enum.MeasurementReference.difference  acceleration_port=false  velocity_port=true  position_port=true  wrap_angle=true  offset=0 rad
  Ideal Torque Sensor : fl_lib/Mechanical/Mechanical Sensors/Ideal Torque Sensor
  Load model : Subsystem  Variant=on
  Mechanical Rotational Reference : fl_lib/Mechanical/Rotational Elements/Mechanical Rotational Reference
  Open Circuit : fl_lib/Electrical/Electrical Elements/Open Circuit  v_specify=off  v_priority=None  v=0 V  v_nominal_specify=off  v_nominal_value=1  v_nominal_unit=V
  PS-Simulink Converter{,1..8} (9 alike) : nesl_utility/PS-Simulink Converter  PhysicalDomain=network_engine_domain  SubClassName=ps_output  LeftPortType=input  RightPortType=output  PseudoPeriodic=off  Frequencies=[]  VectorFormat=inherit  Unit=inherit  AffineConversion=off
  Scope : Scope  Commented=on
  Scope1 : Scope  Commented=on
  SimScape PMSM : ee_lib/Electromechanical/Permanent Magnet/FEM-Parameterized PMSM  parameterization=1  winding_type=ee.enum.statorconnection.wye  iVec=[-2, 0, 2] A  xVec=[0, 20, 40, 60] deg  dfluxdiMatrix=0.0002 * ones(3, 4) Wb/A  dfluxdxMatrix=[0, -.16, .16, 0; 0, -.16, .16, 0; 0, -.16, .16, 0] Wb/rad  calculate_torque_matrix=1  TorqueMatrix=zeros(3, 3, 3, 4) N*m  idVec1=[-200, 0, 200] A  iqVec1=[-200, 0, 200] A  LdMatrix=0.0002 * ones(3, 3) H  LqMatrix=0.0002 * ones(3, 3) H  PmMatrix=0.1 * ones(3, 3) Wb  interp_method=simscape.enum.interpolation.linear  N=6  Rs=interp1(ACloss.n,ACloss.Rac,0) Ohm  Ms=0.00002 H  L0=eMotor.L0 H  loss_param=ee.enum.fem_motor.ironLossesExtended.tabulated3D  losses_oc=[0, 0, 0] W  losses_sc=[0, 0, 0] W  f_losses=60 Hz  Isc_losses=95 A  Inertia=eMotor.J kg*m^2  lam=0 N*m*s/rad  i_d_specify=on  i_d_priority=None  i_d=0 A  i_d_nominal_specify=off  i_d_nominal_value=1  i_d_nominal_unit=A  i_q_specify=on  i_q_priority=None  i_q=0 A  i_q_nominal_specify=off  i_q_nominal_value=1  i_q_nominal_unit=A  torque_specify=on  torque_priority=None  torque=interpn(eMotor.Id,eMotor.Iq,eMotor.th,eMotor.T,0,0,0) N*m  torque_nominal_specify=off  torque_nominal_value=1  torque_nominal_unit=N*m  angular_velocity_specify=on  angular_velocity_priority=High  angular_velocity=0 rpm  angular_velocity_nominal_specify=off  angular_velocity_nominal_value=1  angular_velocity_nominal_unit=rpm  angular_position_specify=on  angular_position_priority=High  angular_position=0 deg  angular_position_nominal_specify=off  angular_position_nominal_value=1  angular_position_nominal_unit=deg  alpha=3.93e-3 1/K  alpha_flux=-0.001 1/K  Tmeas=298.15 K  stator_thermal_mass=100 J/K  stator_initial_temperatures=[298.15, 298.15, 298.15] K  rotor_thermal_mass=200 J/K  rotor_initial_temperature=298.15 K  Rm_percent_rotor=90  Rd_percent_rotor=30  idVec=[-200, 0, 200] A  iqVec=[-200, 0, 200] A  dfluxAdiaMatrix3D=zeros(3, 3, 4) Wb/A  dfluxAdibMatrix3D=zeros(3, 3, 4) Wb/A  dfluxAdicMatrix3D=zeros(3, 3, 4) Wb/A  dfluxAdxMatrix3D=zeros(3, 3, 4) Wb/rad  TorqueMatrix3D=zeros(3, 3, 4) N*m  iaVec=[-200, 0, 200] A  ibVec=[-200, 0, 200] A  icVec=[-200, 0, 200] A  dfluxAdiaMatrix=zeros(3, 3, 3, 4) Wb/A  dfluxAdibMatrix=zeros(3, 3, 3, 4) Wb/A  dfluxAdicMatrix=zeros(3, 3, 3, 4) Wb/A  dfluxAdxMatrix=zeros(3, 3, 3, 4) Wb/rad  param_dq0=ee.enum.fem_motor.fluxTabulationOption.DQcartesian  winding_type_dq0=ee.enum.statorconnection.wye  expose_neutral_port=ee.enum.fem_motor.exposeNeutralPort.yes  nPolePairs=eMotor.p  parks_type=ee.enum.fem_motor.parksType.QleadsD_AphaseToDaxis  idVec2=eMotor.Id A  iqVec2=eMotor.Iq A  magVec2=[0, 100, 200] A  betaVec2=[-180, -90, 0, 90, 180] deg  xVec2=eMotor.th deg  fluxD_dq0=eMotor.Fd Wb  fluxQ_dq0=eMotor.Fq Wb  fluxA_dq0=zeros(3, 3, 7) Wb  Torque_dq0=eMotor.T N*m  fluxD_IBX=zeros(3, 5, 7) Wb  fluxQ_IBX=zeros(3, 5, 7) Wb  fluxA_IBX=zeros(3, 5, 7) Wb  Torque_IBX=zeros(3, 5, 7) N*m  rotorLossCoeff_k_h_DQ=zeros(3, 3) W/Hz  rotorLossCoeff_k_J_DQ=zeros(3, 3) W/Hz^2  rotorLossCoeff_k_ex_DQ=zeros(3, 3) W/Hz^(3/2)  rotorLossCoeff_k_h_IB=zeros(3, 5) W/Hz  rotorLossCoeff_k_J_IB=zeros(3, 5) W/Hz^2  rotorLossCoeff_k_ex_IB=zeros(3, 5) W/Hz^(3/2)  statorLossCoeff_k_h_DQ=zeros(3, 3) W/Hz  statorLossCoeff_k_J_DQ=zeros(3, 3) W/Hz^2  statorLossCoeff_k_ex_DQ=zeros(3, 3) W/Hz^(3/2)  statorLossCoeff_k_h_IB=zeros(3, 5) W/Hz  statorLossCoeff_k_J_IB=zeros(3, 5) W/Hz^2  statorLossCoeff_k_ex_IB=zeros(3, 5) W/Hz^(3/2)  wVec=eMotor.ironLoss.n rpm  rotorLossTable_DQ=eMotor.ironLoss.Pfer W  statorLossTable_DQ=eMotor.ironLoss.Pfes W  rotorLossTable_IB=zeros(3, 5, 2) W  statorLossTable_IB=zeros(3, 5, 2) W  electrical_torque_before_iron_losses_specify=off  electrical_torque_before_iron_losses_priority=None  electrical_torque_before_iron_losses=0 N*m  electrical_torque_before_iron_losses_nominal_specify=off  electrical_torque_before_iron_losses_nominal_value=1  electrical_torque_before_iron_losses_nominal_unit=N*m  Qrotor_specify=off  Qrotor_priority=None  Qrotor=0 J/s  Qrotor_nominal_specify=off  Qrotor_nominal_value=1  Qrotor_nominal_unit=J/s  Qstator_specify=off  Qstator_priority=None  Qstator=0 J/s  Qstator_nominal_specify=off  Qstator_nominal_value=1  Qstator_nominal_unit=J/s
  Voltage Sensor : fl_lib/Electrical/Electrical Sensors/Voltage Sensor
  Voltage Sensor1 : fl_lib/Electrical/Electrical Sensors/Voltage Sensor
  Voltage Sensor2 : fl_lib/Electrical/Electrical Sensors/Voltage Sensor
  abc2dq : Subsystem  Commented=on
  abc2dq1 : Subsystem
  A : PMIOPort  Side=Left
  B : PMIOPort  Port=2  Side=Left
  C : PMIOPort  Port=3  Side=Left
  Iabc : Outport
  thetar : Outport  Port=2
  T : Outport  Port=3
  n_m : Outport  Port=4
  Fdq : Outport  Port=5
  Idq_m : Outport  Port=6
  Vabc : Outport  Port=7
  wires:
  PS-Simulink Converter1/1 -> Bus Creator/2
  Delay/1 -> Bus Creator3/1, thetar/1
  PS-Simulink Converter3/1 -> T/1
  PS-Simulink Converter7/1 -> Gain1/1
  PS-Simulink Converter4/1 -> Bus Creator1/1
  abc2dq1/1(X_dq) -> Idq_m/1
  Constant1/1 -> Bus Creator2/2
  PS-Simulink Converter/1 -> Bus Creator/1
  Gain1/1 -> n_m/1
  Constant/1 -> Bus Creator2/1
  Bus Creator1/1 -> abc2dq/1(Xabc), Vabc/1
  Delay1/1 -> Iabc/1
  PS-Simulink Converter5/1 -> Bus Creator1/2
  PS-Simulink Converter2/1 -> Bus Creator/3
  abc2dq/1(X_dq) -> Scope/1
  Bus Creator2/1 -> Fdq/1
  Bus Creator3/1 -> Scope1/1
  Bus Creator/1 -> abc2dq1/1(Xabc), Delay1/1
  PS-Simulink Converter6/1 -> Bus Creator1/3
  PS-Simulink Converter8/1 -> Bus Creator3/2, Delay/1, abc2dq1/2(theta_r), abc2dq/2(theta_r)
  Tload/1 -> Load model/1(T_ref)
  nload/1 -> Load model/2(n_ref)
  connections:
  C/RConn1 -- Voltage Sensor2/LConn1 -- Current Sensor2/LConn1
  A/RConn1 -- Voltage Sensor/LConn1 -- Current Sensor/LConn1
  Ideal Rotational Motion Sensor/LConn1 -- SimScape PMSM/RConn1 -- Ideal Torque Sensor/LConn1
  B/RConn1 -- Voltage Sensor1/LConn1 -- Current Sensor1/LConn1
  Voltage Sensor/RConn1 -- PS-Simulink Converter4/LConn1
  Current Sensor1/RConn2 -- SimScape PMSM/LConn2
  PS-Simulink Converter3/LConn1 -- Ideal Torque Sensor/RConn2
  Voltage Sensor1/RConn1 -- PS-Simulink Converter5/LConn1
  PS-Simulink Converter1/LConn1 -- Current Sensor1/RConn1
  PS-Simulink Converter/LConn1 -- Current Sensor/RConn1
  Ideal Rotational Motion Sensor/RConn2 -- PS-Simulink Converter7/LConn1
  Current Sensor2/RConn2 -- SimScape PMSM/LConn3
  PS-Simulink Converter8/LConn1 -- Ideal Rotational Motion Sensor/RConn3
  PS-Simulink Converter6/LConn1 -- Voltage Sensor2/RConn1
  PS-Simulink Converter2/LConn1 -- Current Sensor2/RConn1
  Current Sensor/RConn2 -- SimScape PMSM/LConn1
  Voltage Sensor/RConn2 -- Open Circuit/LConn1 -- SimScape PMSM/LConn4 -- Voltage Sensor1/RConn2 -- Voltage Sensor2/RConn2
  SimScape PMSM/RConn2 -- Mechanical Rotational Reference/LConn1 -- Ideal Rotational Motion Sensor/RConn1 -- Load model/LConn2
  Load model/LConn1 -- Ideal Torque Sensor/RConn1

== system Motor_ctrl/Power block - Inverter + Motor/Noncircuital/FM/Mechanical equations ==
  Tload : Inport
  Tm : Inport  Port=2
  RPM : Inport  Port=3
  Constant : Constant  Value=Tf
  Constant1 : Constant  Value=Tv
  Delay One Step1 : Delay  DelayLength=1
  Delay One Step2 : Delay  DelayLength=1
  Gain1 : Gain  Gain=30/pi
  Gain2 : Gain  Gain=Bm  SaturateOnIntegerOverflow=on  OutDataTypeStr=Inherit: Same as input  ParamDataTypeStr=Inherit: Same as input
  Gain3 : Gain  Gain=1/J  SaturateOnIntegerOverflow=on  OutDataTypeStr=Inherit: Same as input  ParamDataTypeStr=Inherit: Same as input
  Gain4 : Gain  Gain=(2*pi)/60
  Integrator : Integrator  InitialCondition=th0  WrapState=on  WrappedStateUpperValue=2*pi  WrappedStateLowerValue=0
  Integrator1 : Integrator
  Integrator2 : Integrator  InitialCondition=th0  WrapState=on  WrappedStateUpperValue=2*pi  WrappedStateLowerValue=0
  Math Function1 : Math  Operator=magnitude^2  SignedPower=on
  Product : Product  SaturateOnIntegerOverflow=on  OutDataTypeStr=Inherit: Same as first input
  Product3 : Product  SaturateOnIntegerOverflow=on  OutDataTypeStr=Inherit: Same as first input
  Product6 : Product  SaturateOnIntegerOverflow=on  OutDataTypeStr=Inherit: Same as first input
  Sign : Signum  ZeroCross=off
  Sum1 : Sum  SaturateOnIntegerOverflow=on  OutDataTypeStr=Inherit: Same as first input
  Sum4 : Sum  SaturateOnIntegerOverflow=on  OutDataTypeStr=Inherit: Same as first input
  Sum5 : Sum  Inputs=--+  SaturateOnIntegerOverflow=on  OutDataTypeStr=Inherit: Same as first input
  Switch : Switch  Criteria=u2 > Threshold  Threshold=2.5  SaturateOnIntegerOverflow=off  InputSameDT=off
  Switch1 : Switch  Criteria=u2 > Threshold  Threshold=2.5  SaturateOnIntegerOverflow=off  InputSameDT=off
  n_m : Outport
  Pmec_out : Outport  Port=2  VectorParamsAs1DForOutWhenUnconnected=off
  thetar : Outport  Port=3
  wires:
  Gain3/1 -> Integrator1/1
  Gain2/1 -> Sum1/2
  Delay One Step2/1 -> Math Function1/1, Sign/1, Gain2/1
  Product6/1 -> Sum1/1
  Sum1/1 -> Sum5/2  "T mech loss"
  Tm/1 -> Delay One Step1/1
  Product/1 -> Pmec_out/1
  Tload/1 -> Sum5/1
  Math Function1/1 -> Product3/2
  Constant1/1 -> Product3/1
  Product3/1 -> Sum4/2
  Constant/1 -> Sum4/1
  Sum5/1 -> Gain3/1
  Sign/1 -> Product6/2
  Sum4/1 -> Product6/1
  Integrator2/1 -> Switch1/3
  Integrator/1 -> Switch1/1
  Switch1/1 -> thetar/1
  Switch/1 -> Gain1/1
  Integrator1/1 -> Integrator/1, Switch/1, Delay One Step2/1, Product/2
  Gain4/1 -> Switch/3, Integrator2/1
  [Ctrl_type] -> Switch/2, Switch1/2
  RPM/1 -> Gain4/1
  Delay One Step1/1 -> Sum5/3, Product/1
  Gain1/1 -> n_m/1

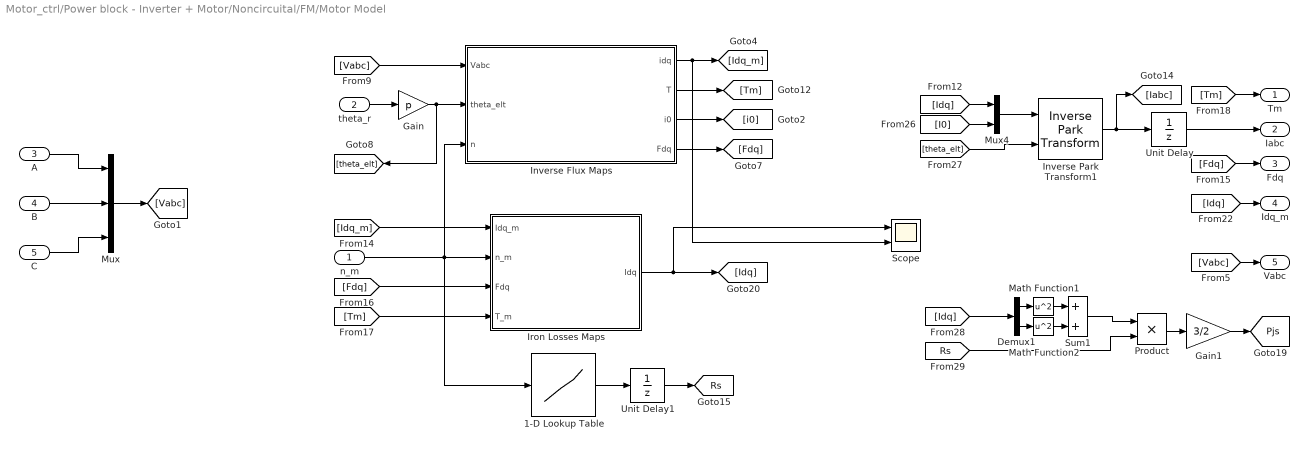
== system Motor_ctrl/Power block - Inverter + Motor/Noncircuital/FM/Motor Model ==
  n_m : Inport
  theta_r : Inport  Port=2
  A : Inport  Port=3
  B : Inport  Port=4
  C : Inport  Port=5
  1-D Lookup Table : Lookup_n-D  NumberOfTableDimensions=1  BreakpointsForDimension1=ACloss.n  Table=ACloss.Rac  InternalRulePriority=Speed  RndMeth=Simplest
  Demux1 : Demux  Outputs=2
  Gain : Gain  Gain=p
  Gain1 : Gain  Gain=3/2
  Inverse Park Transform1 : eeTransforms/Inverse Park Transform  AxisAlignment=D-axis  PowerInvariant=off
  Inverse Flux Maps : Subsystem  Variant=on
  Iron Losses Maps : Subsystem  Variant=on
  Math Function1 : Math  Operator=square
  Math Function2 : Math  Operator=square
  Mux : Mux  Inputs=3
  Mux4 : Mux  Inputs=2
  Product : Product
  Scope : Scope  NumInputPorts=2
  Sum1 : Sum
  Unit Delay : UnitDelay  SampleTime=-1
  Unit Delay1 : UnitDelay  SampleTime=-1
  Tm : Outport
  Iabc : Outport  Port=2
  Fdq : Outport  Port=3
  Idq_m : Outport  Port=4
  Vabc : Outport  Port=5
  tag scope: Pjs=global, Rs=global
  wires:
  Inverse Park Transform1/1 -> [Iabc], Unit Delay/1
  [Idq] -> Idq_m/1
  [Vabc] -> Inverse Flux Maps/1(Vabc)
  [Tm] -> Tm/1
  theta_r/1 -> Gain/1
  [Fdq] -> Fdq/1
  Inverse Flux Maps/2(T) -> [Tm]
  n_m/1 -> Inverse Flux Maps/3(n), 1-D Lookup Table/1, Iron Losses Maps/2(n_m)
  [Fdq] -> Iron Losses Maps/3(Fdq)
  [Tm] -> Iron Losses Maps/4(T_m)
  [Idq_m] -> Iron Losses Maps/1(Idq_m)
  Gain/1 -> [theta_elt], Inverse Flux Maps/2(theta_elt)
  Inverse Flux Maps/3(i0) -> [i0]
  Inverse Flux Maps/4(Fdq) -> [Fdq]
  [Vabc] -> Vabc/1
  [theta_elt] -> Inverse Park Transform1/2
  Mux4/1 -> Inverse Park Transform1/1
  [Idq] -> Mux4/1
  Gain1/1 -> [Pjs]
  Product/1 -> Gain1/1
  [Rs] -> Product/2
  [Idq] -> Demux1/1
  Demux1/1 -> Math Function1/1
  Demux1/2 -> Math Function2/1
  Math Function1/1 -> Sum1/1
  Math Function2/1 -> Sum1/2
  Sum1/1 -> Product/1
  Inverse Flux Maps/1(idq) -> Scope/2, [Idq_m]
  Iron Losses Maps/1(Idq) -> [Idq], Scope/1
  A/1 -> Mux/1
  B/1 -> Mux/2
  C/1 -> Mux/3
  Mux/1 -> [Vabc]
  1-D Lookup Table/1 -> Unit Delay1/1
  Unit Delay/1 -> Iabc/1
  Unit Delay1/1 -> [Rs]
  [I0] -> Mux4/2

== system Motor_ctrl/Power block - Inverter + Motor/Noncircuital/Inverter Model/Inverter Commands ==
  note: 1) Add Subsystem or Model blocks as valid variant choices.
      | 2) You cannot connect blocks at this level. At simulation, connectivity is automatically
      | determined, based on the active variant and port name matching.
  Dabc : Inport
  Enable : Inport  Port=2
  iABC : Inport  Port=3
  Duty : Subsystem  VariantControl=InvModel==0
  PWM : Subsystem  VariantControl=InvModel==1
  Vabc : Outport

== system Motor_ctrl/Power block - Inverter + Motor/Circuital/Inverter Model/Inverter Commands/Duty ==
  Dabc : Inport
  iABC : Inport  Port=2
  Demux : Demux  Outputs=3
  Gain : Gain  Gain=dT/Ts
  Mux14 : Mux  Inputs=6
  Sign : Signum
  Sum : Sum  Inputs=|+-
  X_d1 : Fcn  Expr=1-u(1)
  X_d12 : Fcn  Expr=1-u(1)
  X_d2 : Fcn  Expr=1-u(1)
  G : Outport  VectorParamsAs1DForOutWhenUnconnected=off
  wires:
  iABC/1 -> Sign/1
  Sign/1 -> Gain/1
  Demux/3 -> Mux14/5, X_d2/1
  X_d2/1 -> Mux14/6
  Demux/1 -> X_d12/1, Mux14/1
  Dabc/1 -> Sum/1
  Gain/1 -> Sum/2
  Sum/1 -> Demux/1
  Demux/2 -> Mux14/3, X_d1/1
  X_d1/1 -> Mux14/4
  X_d12/1 -> Mux14/2
  Mux14/1 -> G/1

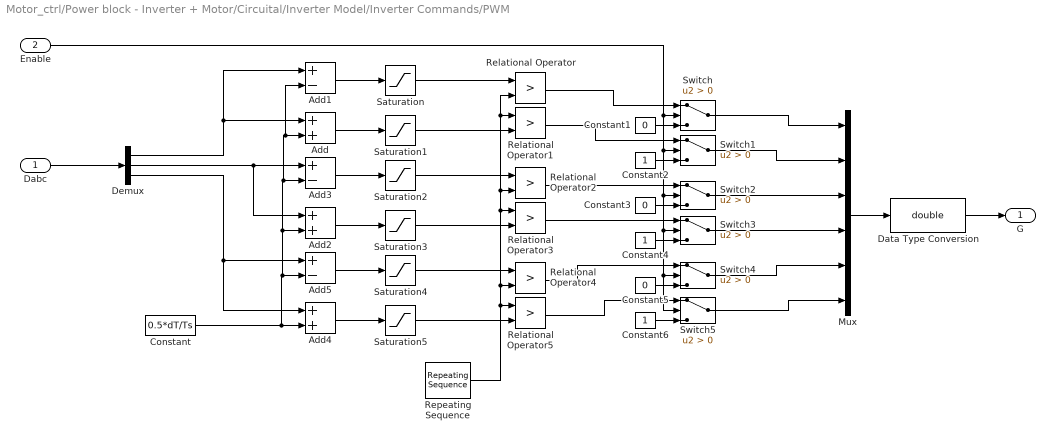
== system Motor_ctrl/Power block - Inverter + Motor/Circuital/Inverter Model/Inverter Commands/PWM ==
  Dabc : Inport
  Enable : Inport  Port=2
  Add : Sum
  Add1 : Sum  Inputs=+-
  Add2 : Sum
  Add3 : Sum  Inputs=+-
  Add4 : Sum
  Add5 : Sum  Inputs=+-
  Constant : Constant  Value=0.5*dT/Ts
  Constant1 : Constant  Value=0
  Constant2 : Constant
  Constant3 : Constant  Value=0
  Constant4 : Constant
  Constant5 : Constant  Value=0
  Constant6 : Constant
  Data Type Conversion : DataTypeConversion  OutDataTypeStr=double  SaturateOnIntegerOverflow=off  RndMeth=Floor
  Demux : Demux  Outputs=3
  Mux : Mux  Inputs=6
  Relational Operator{,1..5} (6 alike) : RelationalOperator  Operator=>  OutDataTypeStr=boolean  RndMeth=Simplest  InputSameDT=off
  Repeating Sequence : simulink/Sources/Repeating Sequence  rep_seq_t=[0 Ts/2 Ts]  rep_seq_y=[1e-6 1-1e-6 1e-6]
  Saturation{,1..5} (6 alike) : Saturate  UpperLimit=1  LowerLimit=0
  Switch{,1..5} (6 alike) : Switch  Criteria=u2 > Threshold  SaturateOnIntegerOverflow=off  InputSameDT=off
  G : Outport
  wires:
  Demux/3 -> Add4/1, Add5/1
  Add4/1 -> Saturation5/1
  Add/1 -> Saturation1/1
  Add5/1 -> Saturation4/1
  Add1/1 -> Saturation/1
  Demux/1 -> Add1/1, Add/1
  Saturation2/1 -> Relational Operator2/1
  Demux/2 -> Add3/1, Add2/1
  Saturation5/1 -> Relational Operator5/2
  Add3/1 -> Saturation2/1
  Add2/1 -> Saturation3/1
  Saturation/1 -> Relational Operator/1
  Saturation4/1 -> Relational Operator4/1
  Saturation1/1 -> Relational Operator1/2
  Saturation3/1 -> Relational Operator3/2
  Dabc/1 -> Demux/1
  Mux/1 -> Data Type Conversion/1
  Repeating Sequence/1 -> Relational Operator/2, Relational Operator1/1, Relational Operator2/2, Relational Operator3/1, Relational Operator4/2, Relational Operator5/1
  Data Type Conversion/1 -> G/1
  Constant/1 -> Add1/2, Add/2, Add3/2, Add2/2, Add5/2, Add4/2
  Relational Operator/1 -> Switch/1
  Constant1/1 -> Switch/3
  Switch/1 -> Mux/1
  Constant2/1 -> Switch1/3
  Switch1/1 -> Mux/2
  Relational Operator1/1 -> Switch1/1
  Constant4/1 -> Switch3/3
  Constant3/1 -> Switch2/3
  Switch2/1 -> Mux/3
  Switch3/1 -> Mux/4
  Relational Operator2/1 -> Switch2/1
  Relational Operator3/1 -> Switch3/1
  Enable/1 -> Switch2/2, Switch4/2, Switch5/2, Switch3/2, Switch1/2, Switch/2
  Constant5/1 -> Switch4/3
  Constant6/1 -> Switch5/3
  Switch4/1 -> Mux/5
  Switch5/1 -> Mux/6
  Relational Operator4/1 -> Switch4/1
  Relational Operator5/1 -> Switch5/1
